simulink model "motor_dtf_antiwindup"  (R2021b)
settings: Solver=FixedStepDiscrete  StartTime=0.0  StopTime=120  RelTol=1e-3
undefined symbols (not defined in the file or in its folder): DiscIntNeverNeededParam
Description:
  | Symmetric FIR Filter
  | This example shows how to use HDL Coder(TM) to check, generate,
  | and verify HDL for a fixed-point symmetric FIR filter.
settings Model: DataTypeOverride=Off  Creator=The MathWorks, Inc.  LastModifiedBy=Marco Milanesi
settings SolverCC: AlgebraicLoopSolver=TrustRegion  AutoInsertRateTranBlk=on
settings DataIOCC: LimitDataPoints=on  SaveFormat=Array  SaveOutput=off  SignalLogging=off  SaveTime=off  ReturnWorkspaceOutputs=off  SignalLoggingName=logsOut
settings OptimizationCC: BlockReduction=off  BooleanDataType=off  ConditionallyExecuteInputs=off  DefaultParameterBehavior=Inlined  InheritOutputTypeSmallerThanSingle=on  InlineInvariantSignals=on  ExpressionDepthLimit=2147483647  InitFltsAndDblsToZero=on  LifeSpan=inf  BufferReusableBoundary=off
settings DebuggingCC: AlgebraicLoopMsg=error  SaveWithParameterizedLinksMsg=none  UnderspecifiedInitializationDetection=Classic  MergeDetectMultiDrivingBlocksExec=none  CheckExecutionContextPreStartOutputMsg=on  SignalResolutionControl=TryResolveAllWithWarning  MultiTaskDSMMsg=warning  MultiTaskCondExecSysMsg=none  SingleTaskRateTransMsg=error  IntegerOverflowMsg=none  ParameterPrecisionLossMsg=none  FcnCallInpInsideContextMsg=warning  BusObjectLabelMismatch=none  StateNameClashWarn=warning  SFUnexpectedBacktrackingDiag=warning  SFNoUnconditionalDefaultTransitionDiag=warning  SFExecutionAtInitializationDiag=none  SFMachineParentedDataDiag=warning  IntegerSaturationMsg=none  ArithmeticOperatorsInVariantConditions=warning
settings HardwareCC: ProdBitPerPointer=32  ProdBitPerSizeT=32  ProdBitPerPtrDiffT=32  ProdLargestAtomicFloat=None  ProdIntDivRoundTo=Undefined  ProdEndianess=Unspecified  ProdWordSize=32  ProdHWDeviceType=ASIC/FPGA  TargetUnknown=on  ProdEqTarget=off
settings ModelReferenceCC: PropagateSignalLabelsOutOfModel=off
settings SFSimCC: SimUseLocalCustomCode=off  CustomCodeUndefinedFunction=UseInterfaceOnly
settings RTWCC: RTWUseLocalCustomCode=off
settings CodeAppCC: StateflowObjectComments=on
settings GRTTargetCC: TargetFcnLib=ansi_tfl_tmw.mat  TargetLangStandard=C89/C90 (ANSI)  CombineOutputUpdateFcns=off  GRTInterface=on
settings ConfigComp: CovMetricSettings=dw  CovSaveCumulativeToWorkspaceVar=on  CovSaveSingleToWorkspaceVar=on  CovExternalEMLEnable=off

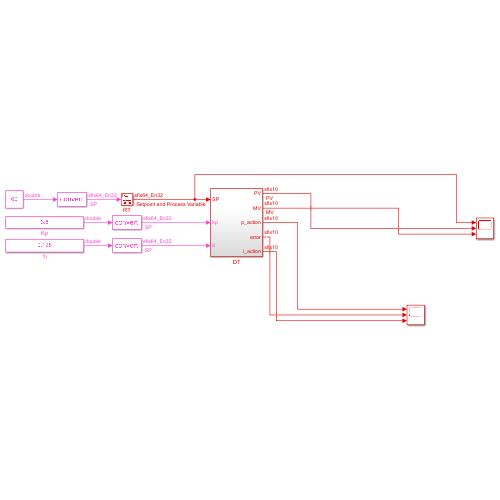
[thumbnail: Simulink's stored preview of the top-level diagram]
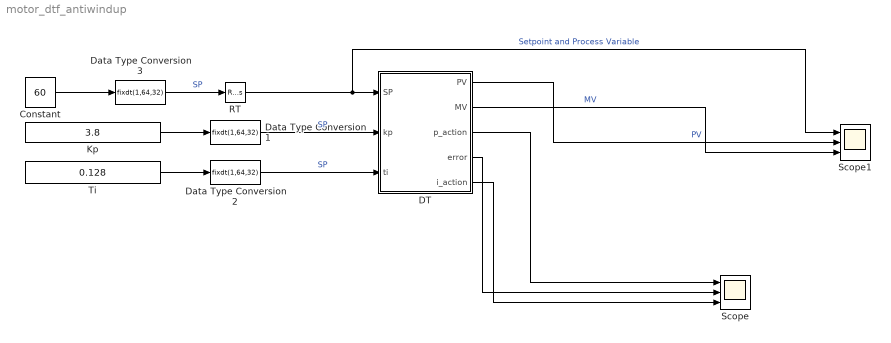
== system motor_dtf_antiwindup ==
  Constant : Constant  Value=60
  DT : Subsystem
  Data Type Conversion1 : DataTypeConversion  OutDataTypeStr=fixdt(1,64,32)
  Data Type Conversion2 : DataTypeConversion  OutDataTypeStr=fixdt(1,64,32)
  Data Type Conversion3 : DataTypeConversion  OutDataTypeStr=fixdt(1,64,32)
  Kp : Constant  Value=3.8
  RT : RateTransition  OutPortSampleTime=0.001
  Scope : Scope  NumInputPorts=3
  Scope1 : Scope  NumInputPorts=3
  Ti : Constant  Value=0.128
  wires:
  Kp/1 -> Data Type Conversion1/1
  Data Type Conversion1/1 -> DT/2(kp)  "SP"
  Data Type Conversion2/1 -> DT/3(ti)  "SP"
  Ti/1 -> Data Type Conversion2/1
  Data Type Conversion3/1 -> RT/1  "SP"
  Constant/1 -> Data Type Conversion3/1
  RT/1 -> Scope1/1, DT/1(SP)  "Setpoint and Process Variable"
  DT/3(p_action) -> Scope/1
  DT/4(error) -> Scope/2
  DT/1(PV) -> Scope1/2  "PV"
  DT/2(MV) -> Scope1/3  "MV"
  DT/5(i_action) -> Scope/3

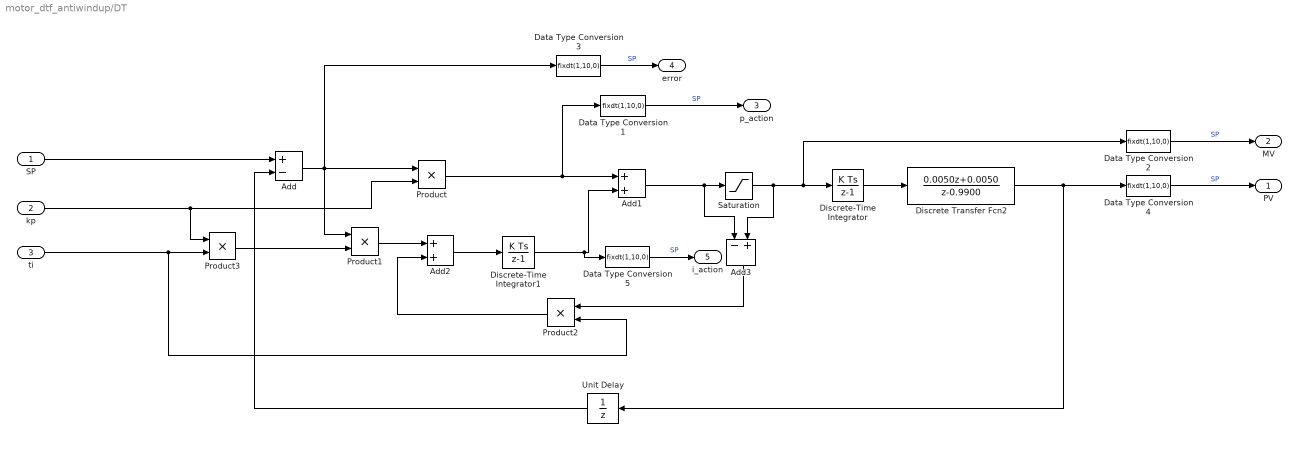
== system motor_dtf_antiwindup/DT ==
  SP : Inport
  kp : Inport  Port=2
  ti : Inport  Port=3
  Add : Sum  Inputs=+-  AccumDataTypeStr=fixdt(1,64,32)  OutDataTypeStr=fixdt(1,64,32)
  Add1 : Sum  AccumDataTypeStr=fixdt(1,64,32)  OutDataTypeStr=fixdt(1,64,32)
  Add2 : Sum  AccumDataTypeStr=fixdt(1,64,32)  OutDataTypeStr=fixdt(1,64,32)
  Add3 : Sum  Inputs=-+  AccumDataTypeStr=fixdt(1,64,32)  OutDataTypeStr=fixdt(1,64,32)
  Data Type Conversion{1..5} (5 alike) : DataTypeConversion  OutDataTypeStr=fixdt(1,10,0)
  Discrete Transfer Fcn2 : DiscreteTransferFcn  Numerator=[0.0050 0.0050]  Denominator=[1 -0.9900]  NumCoefDataTypeStr=fixdt(1,64,32)  DenCoefDataTypeStr=fixdt(1,64,32)  NumProductDataTypeStr=fixdt(1,64,32)  DenProductDataTypeStr=fixdt(1,64,32)  NumAccumDataTypeStr=fixdt(1,64,32)  DenAccumDataTypeStr=fixdt(1,64,32)  OutDataTypeStr=fixdt(1,64,32)
  Discrete-Time Integrator : DiscreteIntegrator  SampleTime=0.001  OutDataTypeStr=fixdt(1,64,32)  ICPrevOutput=DiscIntNeverNeededParam  ICPrevScaledInput=DiscIntNeverNeededParam
  Discrete-Time Integrator1 : DiscreteIntegrator  SampleTime=0.001  OutDataTypeStr=fixdt(1,64,32)  ICPrevOutput=DiscIntNeverNeededParam  ICPrevScaledInput=DiscIntNeverNeededParam
  Product : Product  OutDataTypeStr=fixdt(1,64,32)
  Product1 : Product  OutDataTypeStr=fixdt(1,64,32)
  Product2 : Product  OutDataTypeStr=fixdt(1,64,32)
  Product3 : Product
  Saturation : Saturate  UpperLimit=255  LowerLimit=-255  OutDataTypeStr=fixdt(1,64,32)
  Unit Delay : UnitDelay  SampleTime=0.001  HasFrameUpgradeWarning=on
  PV : Outport  OutDataTypeStr=fixdt(1,10,0)  SampleTime=0.001  VectorParamsAs1DForOutWhenUnconnected=off
  MV : Outport  Port=2  OutDataTypeStr=fixdt(1,10,0)  SampleTime=0.001  VectorParamsAs1DForOutWhenUnconnected=off
  p_action : Outport  Port=3  OutDataTypeStr=fixdt(1,10,0)  SampleTime=0.001  VectorParamsAs1DForOutWhenUnconnected=off
  error : Outport  Port=4  OutDataTypeStr=fixdt(1,10,0)  SampleTime=0.001  VectorParamsAs1DForOutWhenUnconnected=off
  i_action : Outport  Port=5  OutDataTypeStr=fixdt(1,10,0)  SampleTime=0.001  VectorParamsAs1DForOutWhenUnconnected=off
  wires:
  SP/1 -> Add/1
  Discrete Transfer Fcn2/1 -> Data Type Conversion4/1, Unit Delay/1
  Add/1 -> Data Type Conversion3/1, Product/1, Product1/1
  kp/1 -> Product3/1, Product/2
  Product/1 -> Data Type Conversion1/1, Add1/1
  Discrete-Time Integrator1/1 -> Data Type Conversion5/1, Add1/2
  Discrete-Time Integrator/1 -> Discrete Transfer Fcn2/1
  Unit Delay/1 -> Add/2
  Saturation/1 -> Data Type Conversion2/1, Discrete-Time Integrator/1, Add3/2
  Add1/1 -> Add3/1, Saturation/1
  Product1/1 -> Add2/1
  Add2/1 -> Discrete-Time Integrator1/1
  Add3/1 -> Product2/1
  Product2/1 -> Add2/2
  ti/1 -> Product3/2, Product2/2
  Product3/1 -> Product1/2
  Data Type Conversion3/1 -> error/1  "SP"
  Data Type Conversion1/1 -> p_action/1  "SP"
  Data Type Conversion4/1 -> PV/1  "SP"
  Data Type Conversion2/1 -> MV/1  "SP"
  Data Type Conversion5/1 -> i_action/1  "SP"
